simulink model "ex11_state_machines_tb"  (R2023b)
settings: Solver=FixedStepDiscrete  StartTime=0.0  StopTime=100  RelTol=1e-3
settings Model: DataTypeOverride=Off  Creator=foregan  LastModifiedBy=foregan
settings SolverCC: AlgebraicLoopSolver=TrustRegion
settings DataIOCC: LimitDataPoints=on  SaveOutput=off  SaveTime=off
settings OptimizationCC: BlockReduction=off  ConditionallyExecuteInputs=off  DefaultParameterBehavior=Inlined  LifeSpan=inf
settings DebuggingCC: AlgebraicLoopMsg=error  SingleTaskRateTransMsg=error  UnconnectedInputMsg=warning  UnconnectedOutputMsg=warning  UnconnectedLineMsg=warning  AllowSymbolicDim=off  StrictBusMsg=ErrorOnBusTreatedAsVector  SFUnexpectedBacktrackingDiag=warning  SFNoUnconditionalDefaultTransitionDiag=warning  SFExecutionAtInitializationDiag=none  ArithmeticOperatorsInVariantConditions=warning
settings HardwareCC: ProdBitPerPointer=32  ProdBitPerSizeT=32  ProdBitPerPtrDiffT=32  ProdLargestAtomicFloat=None  ProdIntDivRoundTo=Undefined  ProdEndianess=Unspecified  ProdWordSize=32  ProdHWDeviceType=ASIC/FPGA->ASIC/FPGA  ProdEqTarget=off
settings ModelReferenceCC: EnableRefExpFcnMdlSchedulingChecks=on
settings SFSimCC: SimUseLocalCustomCode=off  CustomCodeUndefinedFunction=UseInterfaceOnly
settings RTWCC: RTWUseLocalCustomCode=off
settings CodeAppCC: StateflowObjectComments=on
settings GRTTargetCC: TargetLangStandard=C89/C90 (ANSI)
settings ConfigComp: CovScope=ReferencedModels  CovMetricSettings=dw  CovSaveCumulativeToWorkspaceVar=on  CovSaveSingleToWorkspaceVar=on  CovExternalEMLEnable=off  CovSFcnEnable=off

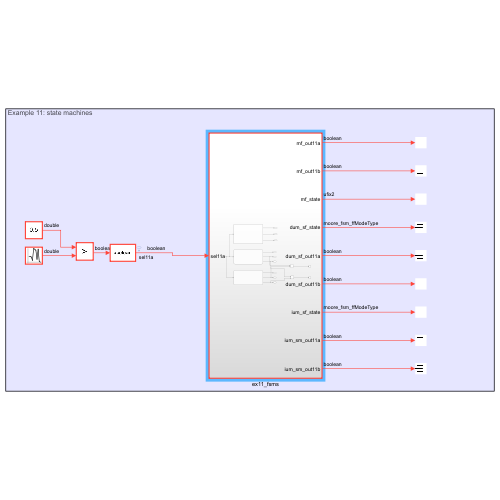
[thumbnail: Simulink's stored preview of the top-level diagram]
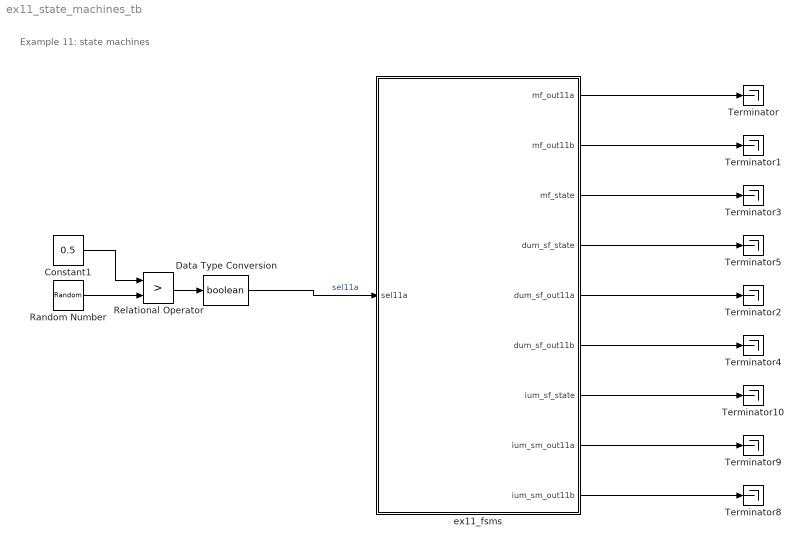
== system ex11_state_machines_tb ==
  note: Example 11: state machines
  Constant1 : Constant  Value=0.5  SampleTime=1
  Data Type Conversion : DataTypeConversion  OutDataTypeStr=boolean  SaturateOnIntegerOverflow=off  RndMeth=Floor
  Random Number : RandomNumber  SampleTime=1
  Relational Operator : RelationalOperator  Operator=>  OutDataTypeStr=boolean  RndMeth=Simplest  InputSameDT=off
  Terminator{,1..5,8..10} (9 alike) : Terminator
  ex11_fsms : Subsystem
  wires:
  ex11_fsms/8(ium_sm_out11a) -> Terminator9/1
  ex11_fsms/9(ium_sm_out11b) -> Terminator8/1
  ex11_fsms/7(ium_sf_state) -> Terminator10/1
  Data Type Conversion/1 -> ex11_fsms/1(sel11a)  "sel11a"
  ex11_fsms/1(mf_out11a) -> Terminator/1
  ex11_fsms/2(mf_out11b) -> Terminator1/1
  Relational Operator/1 -> Data Type Conversion/1
  ex11_fsms/3(mf_state) -> Terminator3/1
  ex11_fsms/6(dum_sf_out11b) -> Terminator4/1
  Random Number/1 -> Relational Operator/2
  ex11_fsms/5(dum_sf_out11a) -> Terminator2/1
  ex11_fsms/4(dum_sf_state) -> Terminator5/1
  Constant1/1 -> Relational Operator/1

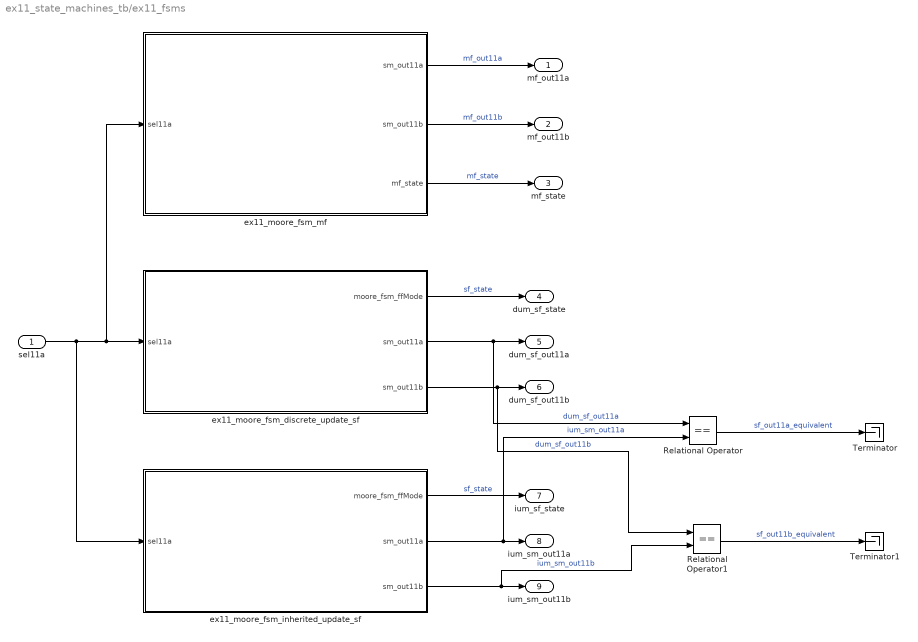
== system ex11_state_machines_tb/ex11_fsms ==
  sel11a : Inport
  Relational Operator : RelationalOperator  Operator===  OutDataTypeStr=boolean  RndMeth=Simplest  InputSameDT=off
  Relational Operator1 : RelationalOperator  Operator===  OutDataTypeStr=boolean  RndMeth=Simplest  InputSameDT=off
  Terminator : Terminator
  Terminator1 : Terminator
  ex11_moore_fsm_discrete_update_sf : Stateflow chart  TreatAsAtomicUnit=on
  ex11_moore_fsm_inherited_update_sf : Stateflow chart  TreatAsAtomicUnit=on
  ex11_moore_fsm_mf : MATLAB Function  TreatAsAtomicUnit=on
  mf_out11a : Outport
  mf_out11b : Outport  Port=2
  mf_state : Outport  Port=3
  dum_sf_state : Outport  Port=4
  dum_sf_out11a : Outport  Port=5
  dum_sf_out11b : Outport  Port=6
  ium_sf_state : Outport  Port=7
  ium_sm_out11a : Outport  Port=8
  ium_sm_out11b : Outport  Port=9
  wires:
  ex11_moore_fsm_discrete_update_sf/2(sm_out11a) -> Relational Operator/1, dum_sf_out11a/1  "dum_sf_out11a"
  ex11_moore_fsm_mf/1(sm_out11a) -> mf_out11a/1  "mf_out11a"
  ex11_moore_fsm_mf/2(sm_out11b) -> mf_out11b/1  "mf_out11b"
  ex11_moore_fsm_mf/3(mf_state) -> mf_state/1  "mf_state"
  ex11_moore_fsm_discrete_update_sf/3(sm_out11b) -> Relational Operator1/1, dum_sf_out11b/1  "dum_sf_out11b"
  ex11_moore_fsm_discrete_update_sf/1(moore_fsm_ffMode) -> dum_sf_state/1  "sf_state"
  ex11_moore_fsm_inherited_update_sf/3(sm_out11b) -> Relational Operator1/2, ium_sm_out11b/1  "ium_sm_out11b"
  ex11_moore_fsm_inherited_update_sf/2(sm_out11a) -> Relational Operator/2, ium_sm_out11a/1  "ium_sm_out11a"
  ex11_moore_fsm_inherited_update_sf/1(moore_fsm_ffMode) -> ium_sf_state/1  "sf_state"
  sel11a/1 -> ex11_moore_fsm_inherited_update_sf/1(sel11a), ex11_moore_fsm_mf/1(sel11a), ex11_moore_fsm_discrete_update_sf/1(sel11a)
  Relational Operator/1 -> Terminator/1  "sf_out11a_equivalent"
  Relational Operator1/1 -> Terminator1/1  "sf_out11b_equivalent"

== stateflow chart ex11_state_machines_tb/ex11_fsms/ex11_moore_fsm_inherited_update_sf ==
  settings: sampleTime=1  stateMachineType=MOORE_MACHINE  executeAtInitialization=1
  state IDLE
    sm_out11a = true;
    sm_out11b = false;
  state ACTIVE2
    sm_out11a = false;
    sm_out11b = false;
  state ACTIVE1
    sm_out11a = true;
    sm_out11b = true;
  (default) -> IDLE
  ACTIVE2 -> IDLE : [sel11a]
  IDLE -> ACTIVE1 : [sel11a]
  ACTIVE1 -> ACTIVE2 : [sel11a]
  data: moore_fsm_ffMode output Enum: moore_fsm_ffModeType; sel11a input; sm_out11a output; sm_out11b output

== stateflow chart ex11_state_machines_tb/ex11_fsms/ex11_moore_fsm_discrete_update_sf ==
  settings: updateMethod=DISCRETE  sampleTime=1  stateMachineType=MOORE_MACHINE  executeAtInitialization=1
  state IDLE
    sm_out11a = true;
    sm_out11b = false;
  state ACTIVE2
    sm_out11a = false;
    sm_out11b = false;
  state ACTIVE1
    sm_out11a = true;
    sm_out11b = true;
  (default) -> IDLE
  ACTIVE2 -> IDLE : [sel11a]
  IDLE -> ACTIVE1 : [sel11a]
  ACTIVE1 -> ACTIVE2 : [sel11a]
  data: moore_fsm_ffMode output Enum: moore_fsm_ffModeType; sel11a input; sm_out11a output; sm_out11b output

== matlab function ex11_state_machines_tb/ex11_fsms/ex11_moore_fsm_mf ==
  settings: fimath=|
      | fimath(...
      | 'RoundMode', 'nearest',...
      | 'OverflowMode', 'saturate',...
      | 'ProductMode', 'FullPrecision', 'ProductWordLength', 128,...
      | 'SumMode', 'FullPrecision', 'SumWordLength', 128,...
      | 'CastBeforeSum', true)
  data: sm_out11a output; sel11a input; sm_out11b output boolean size=1; mf_state output
function [sm_out11a, sm_out11b, mf_state] = fcn(sel11a)

persistent moore_state_reg;
if isempty(moore_state_reg)
    moore_state_reg = fi(0, 0, 2, 0);
end

IDLE = 0;
ACTIVE1 = 1;
ACTIVE2 = 2;

switch (moore_state_reg(1))

    case IDLE
        sm_out11a = true;
        sm_out11b = false;
        mf_state = moore_state_reg(1);

        if (~sel11a)
            moore_state_reg(1) = IDLE;
        else
            moore_state_reg(1) = ACTIVE1;
        end

    case ACTIVE1

        sm_out11a = true;
        sm_out11b = true;
        mf_state = moore_state_reg(1);

        if (~sel11a)
            moore_state_reg(1) = ACTIVE1;
        else
            moore_state_reg(1) = ACTIVE2;
        end

    case ACTIVE2
        sm_out11a = false;
        sm_out11b = false;
        mf_state = moore_state_reg(1);

        if (~sel11a)
            moore_state_reg(1) = ACTIVE2;
        else
            moore_state_reg(1) = IDLE;
        end

    otherwise
        mf_state = moore_state_reg(1);
        sm_out11a = false;
        sm_out11b = false;
end
